simulink model "pulsesteppermotor2"  (R2019a)
settings: Solver=FixedStepAuto  StartTime=0.0  StopTime=100  RelTol=1e-3  EnableMultiTasking=on
libraries: arduinolib x3
settings Model: EnablePacing=on  ExtModeTrigDuration=2  Creator=ADMIN  LastModifiedBy=ADMIN
settings OptimizationCC: EnhancedBackFolding=on  PassReuseOutputArgsAs=Individual arguments  MaxStackSize=64  OptimizeBlockOrder=speed  DifferentSizesBufferReuse=on  OptimizationCustomize=off
settings DebuggingCC: ParameterTunabilityLossMsg=error
settings HardwareCC: ProdBitPerInt=16  ProdBitPerPointer=16  ProdBitPerSizeT=16  ProdBitPerPtrDiffT=16  ProdLargestAtomicFloat=None  ProdWordSize=8  ProdHWDeviceType=Atmel->AVR
settings SFSimCC: MATLABDynamicMemAlloc=off
settings RTWCC: SystemTargetFile=ert.tlc  HardwareBoard=Arduino Uno  TLCOptions=-aInlineSetEventsForThisBaseRateFcn=TLC_FALSE -aSuppressMultiTaskScheduler=TLC_FALSE -aRateBasedStepFcn=1  TemplateMakefile=ert_default_tmf  GenerateReport=on  Toolchain=Arduino AVR  BuildConfiguration=Faster Runs  IncludeHyperlinkInReport=on  LaunchReport=on  GenerateTraceInfo=on  GenerateTraceReport=on  GenerateTraceReportSl=on  GenerateTraceReportSf=on  GenerateTraceReportEml=on
settings CodeAppCC: ForceParamTrailComments=on  IgnoreCustomStorageClasses=off  OperatorAnnotations=on  SimulinkDataObjDesc=on  SFDataObjDesc=on  InsertBlockDesc=on
settings ERTTargetCC: SupportContinuousTime=on  SupportVariableSizeSignals=on  ExtModeStaticAllocSize=250

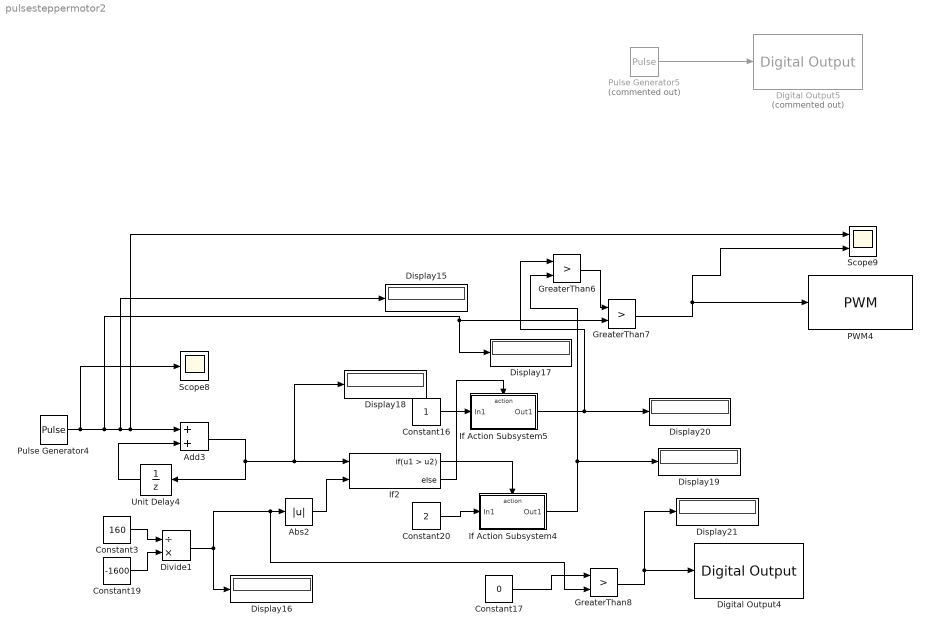
== system pulsesteppermotor2 ==
  Abs2 : Abs
  Add3 : Sum
  Constant16 : Constant
  Constant17 : Constant  Value=0
  Constant19 : Constant  Value=-1600
  Constant20 : Constant  Value=2
  Constant3 : Constant  Value=160
  Digital Output4 : arduinolib/Digital Output  pinNumber=8  blockPlatform=arduino
  Digital Output5 : arduinolib/Digital Output  Commented=on  pinNumber=9  blockPlatform=arduino
  Display{15..21} (7 alike) : Display
      settings: Format=decimal (Stored Integer)
  Divide1 : Product  Inputs=/*
  GreaterThan6 : RelationalOperator  Operator=>  OutDataTypeStr=fixdt(1,16)  RndMeth=Simplest
  GreaterThan7 : RelationalOperator  Operator=>  OutDataTypeStr=fixdt(1,16)  RndMeth=Simplest
  GreaterThan8 : RelationalOperator  Operator=>  OutDataTypeStr=fixdt(1,16)  RndMeth=Simplest
  If Action Subsystem4 : Subsystem  TreatAsAtomicUnit=on
  If Action Subsystem5 : Subsystem  TreatAsAtomicUnit=on
  If2 : If  NumInputs=2  IfExpression=u1 > u2
  PWM4 : arduinolib/PWM  pinNumber=10  EnableInputFrequency=off  InitialFrequency=2000  InitialDutyCycle=0  NotificationType=None  blockPlatform=arduino
  Pulse Generator4 : DiscretePulseGenerator  PulseType=Time based  Amplitude=0.1  Period=0.44  PulseWidth=50
  Pulse Generator5 : DiscretePulseGenerator  Commented=on  PulseType=Time based  Period=0.0000001  PulseWidth=50
  Scope8 : Scope
  Scope9 : Scope  NumInputPorts=2
  Unit Delay4 : UnitDelay  SampleTime=-1  HasFrameUpgradeWarning=on
  wires:
  Constant17/1 -> GreaterThan8/1
  GreaterThan8/1 -> Display21/1, Digital Output4/1
  Abs2/1 -> If2/2
  GreaterThan7/1 -> PWM4/1, Scope9/2
  If Action Subsystem4/1(Out1) -> Display19/1, GreaterThan6/2
  If Action Subsystem5/1(Out1) -> Display20/1, GreaterThan6/1
  Constant16/1 -> If Action Subsystem5/1(In1)
  Pulse Generator4/1 -> Scope8/1, GreaterThan7/2, Display17/1, Display15/1, Scope9/1, Add3/1
  If2/2 -> If Action Subsystem5/Action
  GreaterThan6/1 -> GreaterThan7/1
  Constant20/1 -> If Action Subsystem4/1(In1)
  Unit Delay4/1 -> Add3/2
  Divide1/1 -> Display16/1, GreaterThan8/2, Abs2/1
  If2/1 -> If Action Subsystem4/Action
  Add3/1 -> Unit Delay4/1, Display18/1, If2/1
  Constant19/1 -> Divide1/2
  Constant3/1 -> Divide1/1
  Pulse Generator5/1 -> Digital Output5/1

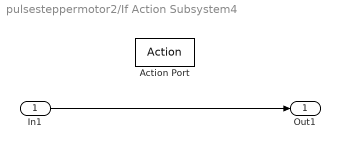
== system pulsesteppermotor2/If Action Subsystem4 ==
  In1 : Inport
  Action Port : ActionPort  ActionPortLabel=if(u1 > u2)
  Out1 : Outport
  wires:
  In1/1 -> Out1/1

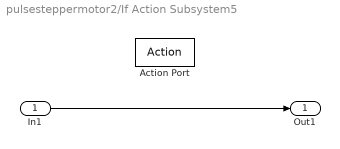
== system pulsesteppermotor2/If Action Subsystem5 ==
  In1 : Inport
  Action Port : ActionPort  ActionPortLabel=else
  Out1 : Outport
  wires:
  In1/1 -> Out1/1
